simulink subsystem "windModel"  (R2026a)
settings: Solver=VariableStepAuto
values from neighbouring files (symbols this model uses):
  windParams = 0.0    [plantParams.sldd]
undefined symbols (not defined in the file or in its folder): F, Light, MIL
libraries: aerolibwind2 x2
settings Model: DataDictionary=plantParams.sldd  EnableAccessToBaseWorkspace=off  Creator=nathanwu  LastModifiedBy=maxhu

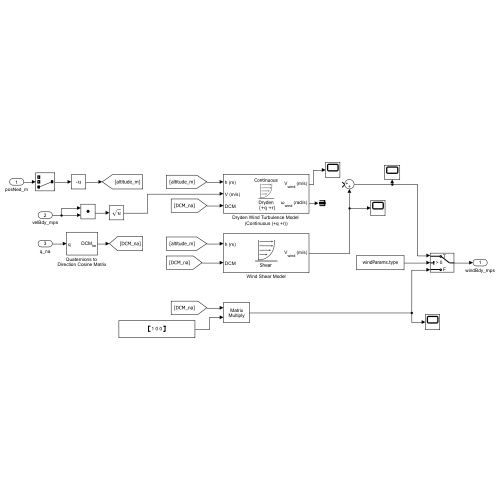
[thumbnail: Simulink's stored preview of the top-level diagram]
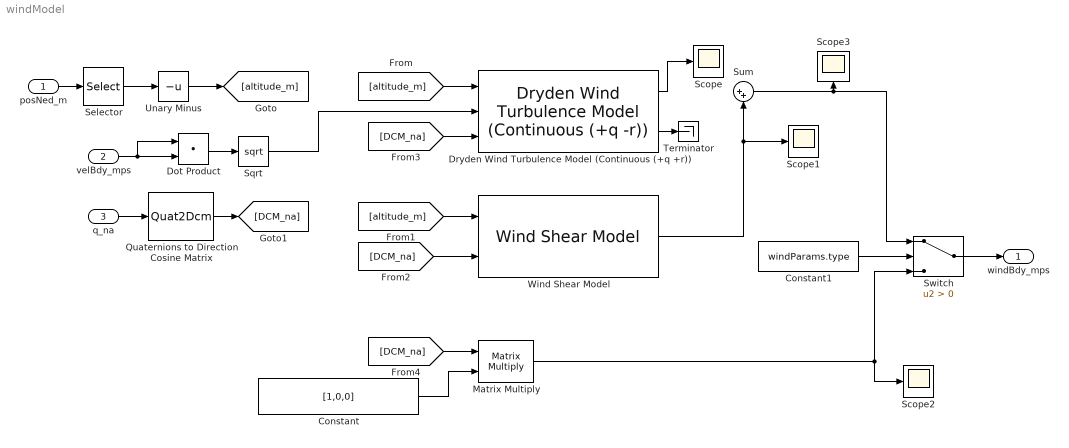
== system windModel ==
  posNed_m : Inport
  velBdy_mps : Inport  Port=2
  q_na : Inport  Port=3
  Constant : Constant  Value=[1,0,0]
  Constant1 : Constant  Value=windParams.type
  Dot Product : DotProduct  OutDataTypeStr=Inherit: Inherit via internal rule
  Dryden Wind Turbulence Model (Continuous (+q +r)) : aerolibwind2/Dryden Wind Turbulence Model  (Continuous (+q -r))  units=Metric (MKS)  spec=MIL-F-8785C  model=Continuous Dryden (+q +r)  W20=15  Wdeg=0  TurbProb=10^-2 - Light  L_high=533.4  Wingspan=10  ts=0.1  Seed=[23341 23342 23343 23344]  T_on=on
      settings: LibrarySourceBlock=|
      | aerolibwind2/Dryden Wind Turbulence Model
      | (Continuous (+q +r))
  Matrix Multiply : Product  Multiplication=Matrix(*)
  Quaternions to Direction Cosine Matrix : Quat2Dcm
  Scope{,1..3} (4 alike) : Scope
      Scope settings: ActiveDisplayYMinimum=-4.511373180461316  ActiveDisplayYMaximum=4.2619597588138483  DataLoggingVariableName=ScopeData6
      Scope1 settings: DataLoggingVariableName=ScopeData9
      Scope2 settings: ActiveDisplayYMinimum=-1  ActiveDisplayYMaximum=1  DataLoggingVariableName=ScopeData10
      Scope3 settings: DataLoggingVariableName=ScopeData11
  Selector : Selector  InputPortWidth=3  IndexOptions=Index vector (dialog)  Indices=3  OutputSizes=1
  Sqrt : Sqrt
  Sum : Sum  Inputs=|++
  Switch : Switch  Criteria=u2 > Threshold  SaturateOnIntegerOverflow=off  InputSameDT=off
  Terminator : Terminator
  Unary Minus : UnaryMinus
  Wind Shear Model : aerolibwind2/Wind Shear Model  units=Metric (MKS)  phase=Category C - Terminal Flight Phase  W_20=15  Wdeg=0
  windBdy_mps : Outport
  wires:
  velBdy_mps/1 -> Dot Product/1, Dot Product/2
  Wind Shear Model/1 -> Sum/2, Scope1/1
  Sqrt/1 -> Dryden Wind Turbulence Model (Continuous (+q +r))/2
  Dryden Wind Turbulence Model (Continuous (+q +r))/2 -> Terminator/1
  [DCM_na] -> Dryden Wind Turbulence Model (Continuous (+q +r))/3
  q_na/1 -> Quaternions to Direction Cosine Matrix/1
  [altitude_m] -> Dryden Wind Turbulence Model (Continuous (+q +r))/1
  [altitude_m] -> Wind Shear Model/1
  Unary Minus/1 -> [altitude_m]
  posNed_m/1 -> Selector/1
  Selector/1 -> Unary Minus/1
  Dot Product/1 -> Sqrt/1
  Quaternions to Direction Cosine Matrix/1 -> [DCM_na]
  [DCM_na] -> Matrix Multiply/1
  Constant/1 -> Matrix Multiply/2
  Matrix Multiply/1 -> Switch/3, Scope2/1
  Constant1/1 -> Switch/2
  [DCM_na] -> Wind Shear Model/2
  Dryden Wind Turbulence Model (Continuous (+q +r))/1 -> Scope/1
  Switch/1 -> windBdy_mps/1
  Sum/1 -> Scope3/1, Switch/1
